simulink model "Engine_harness_model"  (R2021a)
settings: Solver=daessc  StartTime=0.0  StopTime=60*10  RelTol=1e-3  AbsTol=1e-3
PreLoadFcn:
  | Engine_harness_setup
undefined symbols (not defined in the file): engine
libraries: fl_lib x7, nesl_utility x5
settings Model: Creator=isaacito  LastModifiedBy=isaacito
settings DataIOCC: ReturnWorkspaceOutputs=off
settings DebuggingCC: UnconnectedInputMsg=none  UnconnectedOutputMsg=none  UnconnectedLineMsg=none
settings RTWCC: DLArmComputeVersion=20.02.1
settings SimscapeCC: SimscapeLogType=all  SimscapeLogSimulationStatistics=on  SimscapeLogLimitData=off

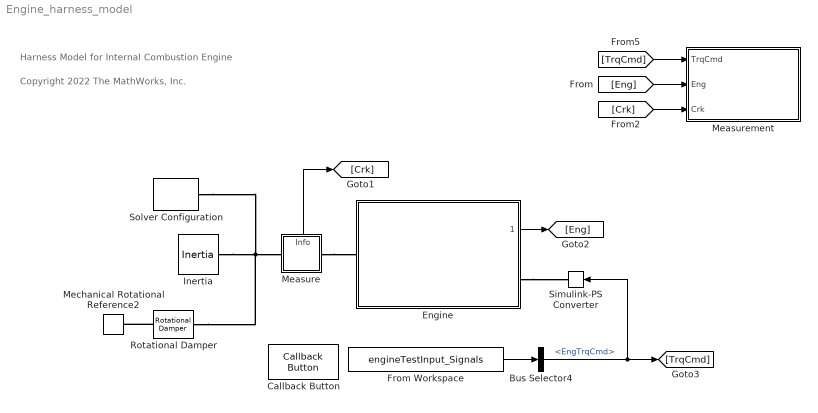
== system Engine_harness_model ==
  note: Copyright 2022 The MathWorks, Inc.
  note: Harness Model for Internal Combustion Engine
  Bus Selector4 : BusSelector  OutputSignals=EngTrqCmd
  Callback Button : CallbackButton  ButtonText=Plot input
      settings: ClickFcn="Engine_plot_inputs_simple(\"engineTestInput_Signals\")"
  Engine : Subsystem  ReferencedSubsystem=EngineCustom_refsub
  From Workspace : FromWorkspace  VariableName=engineTestInput_Signals  OutDataTypeStr=Bus: engineTestInput_Bus  OutputAfterFinalValue=Holding final value
      settings: AttributesFormatString=|
      | %<OutDataTypeStr>
      | Interpolate: %<Interpolate>
  Inertia : fl_lib/Mechanical/Rotational Elements/Inertia  inertia=engine.inertia_kg_m2 kg*m^2  num_ports=foundation.enum.numPorts2.one  w_specify=on  w_priority=High  w=initial.engine_speed_rpm rpm  w_nominal_specify=off  w_nominal_unit=rad/s  w_nominal_value=1  t_specify=off  t_priority=None  t=0 N*m  t_nominal_specify=off  t_nominal_unit=N*m  t_nominal_value=1
      settings: SourceProductBaseCode=PW,SS,VE
      settings: AttributesFormatString=|
      | Initial: %<w> [%<w_unit>]
      | Priority: %<w_priority>
  Measure : Subsystem
      settings: PortSchema="{\"entries\":[{\"content\":{\"sides\":[{\"content\":{\"connectorIds\":[\"LConn1\"]},\"type\":\"ConnectorPlacement.EquallySpacedRectSide\",\"uuid\":\"07c3a1fd-7b75-413d-9cf1-ab8270959579\"},{\"content\":{\"connectorIds\":[\"RConn1\"],\"side\":\"RIGHT\"},\"type\":\"ConnectorPlacement.EquallySpacedRectSide\",\"uuid\":\"82fb53da-addd-4028-9f33-7d5a40e2d331\"},{\"content\":{\"connectorIds\":[],\"side\":\"TOP\"},\"type\":\"ConnectorPlacement.EquallySpacedRectSide\",\"uuid\":\"88b61019-5b08-4fd4-81f8-a447296a1b8b\"},{\"content\":{\"connectorIds\":[\"Out1\"],\"side\":\"BOTTOM\"},\"type\":\"ConnectorPlacement.EquallySpacedRectSide\",\"uuid\":\"d19d7c6f-4100-43ea-b025-020464ef54d5\"}]},\"type\":\"ConnectorPlacement.EquallySpacedConnector\",\"uuid\":\"a316222e-f9ce-4776-9d48-54bd569192f1\"}],\"packageUris\":[\"http://schema.mathworks.com/mf0/Connector/R2020b\"],\"version\":\"1.0\"}"
  Measurement : Subsystem
  Mechanical Rotational Reference2 : fl_lib/Mechanical/Rotational Elements/Mechanical Rotational Reference
      settings: SourceProductBaseCode=PW,SS,VE
  Rotational Damper : fl_lib/Mechanical/Rotational Elements/Rotational Damper  D=engine.damping_Nm_per_rpm m*N/rpm  w_specify=off  w_priority=None  w=0 rad/s  w_nominal_specify=off  w_nominal_unit=rad/s  w_nominal_value=1  t_specify=off  t_priority=None  t=0 N*m  t_nominal_specify=off  t_nominal_unit=N*m  t_nominal_value=1
      settings: SourceProductBaseCode=PW,SS,VE
  Simulink-PS Converter : nesl_utility/Simulink-PS Converter  PhysicalDomain=network_engine_domain  SubClassName=ps_input  LeftPortType=input  RightPortType=output  PseudoPeriodic=off  Frequencies=[]  NoiseDistribution=none  NoiseParameters=[]  Unit=N*m  AffineConversion=off  FilteringAndDerivatives=provide  SimscapeFilterOrder=1  InputFilterTimeConstant=0.001  UdotUserProvided=0
      settings: SourceProductBaseCode=SS,PW,VE
  Solver Configuration : nesl_utility/Solver Configuration  PhysicalDomain=network_engine_domain  SubClassName=solver  LeftPortType=input  RightPortType=generic  Tones=[]  Harmonics=[]  SimulateNoise=off  Profile=off  UseLocalSampling=off  EnableSwitchedLinearOptims=on  FrequencyDomain=off  UseCCode=off  RelTol=0.001  AbsTol=0.001  MinStep=1e-09  ToWorkspace=off  RevertToSquareIcSolve=off  NumHomotopyIterations=100  PhasorMode=off  PhasorModeNumHarmonics=1  DoDC=off  ResidualTolerance=1e-09  UseLocalSolver=off  LocalSolverChoice=NE_BACKWARD_EULER_ADVANCER  LocalSolverSampleTime=0.001  DoFixedCost=off  MaxNonlinIter=3  MaxModeIter=2  ComputeImpulses=off  ImpulseIterations=2  LinearAlgebra=auto  EquationFormulation=NE_TIME_EF  DelaysMemoryBudget=1024  AutomaticFiltering=on  FilteringTimeConstant=0.001  PartitionStorageMethod=AS_NEEDED  PartitionMemoryBudget=1024  PartitionMethod=ROBUST
      settings: AttributesFormatString=Local solver: %<UseLocalSolver>  SourceProductBaseCode=SS,PW,VE
  wires:
  From Workspace/1 -> Bus Selector4/1
  Bus Selector4/1 -> [TrqCmd], Simulink-PS Converter/1  "<EngTrqCmd>"
  Engine/1 -> [Eng]
  Measure/1(Info) -> [Crk]
  [TrqCmd] -> Measurement/1(TrqCmd)
  [Eng] -> Measurement/2(Eng)
  [Crk] -> Measurement/3(Crk)
  connections:
  Rotational Damper/RConn1 -- Mechanical Rotational Reference2/LConn1
  Inertia/LConn1 -- Solver Configuration/RConn1 -- Rotational Damper/LConn1 -- Measure/RConn1
  Engine/RConn1 -- Simulink-PS Converter/RConn1
  Measure/LConn1 -- Engine/LConn1

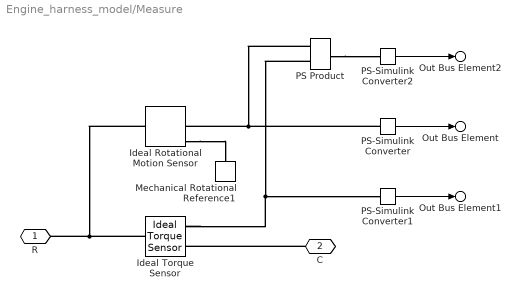
== system Engine_harness_model/Measure ==
  Ideal Rotational Motion Sensor : fl_lib/Mechanical/Mechanical Sensors/Ideal Rotational Motion Sensor  wrap_angle=simscape.enum.onoff.off  offset=0 rad
      settings: SourceProductBaseCode=PW,SS,VE
  Ideal Torque Sensor : fl_lib/Mechanical/Mechanical Sensors/Ideal Torque Sensor
      settings: SourceProductBaseCode=PW,SS,VE
  Mechanical Rotational Reference1 : fl_lib/Mechanical/Rotational Elements/Mechanical Rotational Reference
      settings: SourceProductBaseCode=PW,SS,VE
  PS Product : fl_lib/Physical Signals/Functions/PS Product
  PS-Simulink Converter : nesl_utility/PS-Simulink Converter  PhysicalDomain=network_engine_domain  SubClassName=ps_output  LeftPortType=input  RightPortType=output  PseudoPeriodic=off  Frequencies=[]  Unit=rpm  AffineConversion=off
      settings: SourceProductBaseCode=SS,PW,VE
  PS-Simulink Converter1 : nesl_utility/PS-Simulink Converter  PhysicalDomain=network_engine_domain  SubClassName=ps_output  LeftPortType=input  RightPortType=output  PseudoPeriodic=off  Frequencies=[]  Unit=N*m  AffineConversion=off
      settings: SourceProductBaseCode=SS,PW,VE
  PS-Simulink Converter2 : nesl_utility/PS-Simulink Converter  PhysicalDomain=network_engine_domain  SubClassName=ps_output  LeftPortType=input  RightPortType=output  PseudoPeriodic=off  Frequencies=[]  Unit=kW  AffineConversion=off
      settings: SourceProductBaseCode=SS,PW,VE
  R : PMIOPort  Side=Left
  C : PMIOPort  Port=2  Side=Right
  Out Bus Element : Outport  PortName=Info  Element=CrkSpd
  Out Bus Element1 : Outport  PortName=Info  Element=CrkTrq
  Out Bus Element2 : Outport  PortName=Info  Element=CrkPwr
  wires:
  PS-Simulink Converter/1 -> Out Bus Element/1
  PS-Simulink Converter1/1 -> Out Bus Element1/1
  PS-Simulink Converter2/1 -> Out Bus Element2/1
  connections:
  PS-Simulink Converter/LConn1 -- PS Product/LConn1 -- Ideal Rotational Motion Sensor/RConn2
  Ideal Rotational Motion Sensor/RConn1 -- Mechanical Rotational Reference1/LConn1
  Ideal Torque Sensor/RConn2 -- PS Product/LConn2 -- PS-Simulink Converter1/LConn1
  Ideal Torque Sensor/LConn1 -- R/RConn1 -- Ideal Rotational Motion Sensor/LConn1
  C/RConn1 -- Ideal Torque Sensor/RConn1
  PS Product/RConn1 -- PS-Simulink Converter2/LConn1

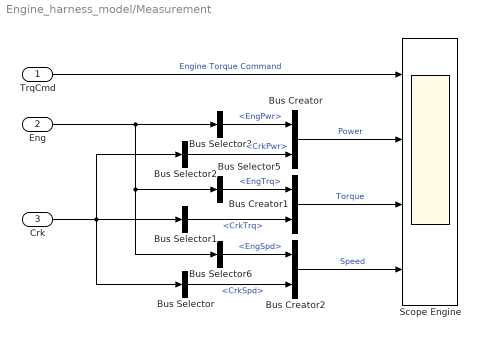
== system Engine_harness_model/Measurement ==
  TrqCmd : Inport
  Eng : Inport  Port=2
  Crk : Inport  Port=3
  Bus Creator : BusCreator  Inputs=2
  Bus Creator1 : BusCreator  Inputs=2
  Bus Creator2 : BusCreator  Inputs=2
  Bus Selector : BusSelector  OutputSignals=CrkSpd
  Bus Selector1 : BusSelector  OutputSignals=CrkTrq
  Bus Selector2 : BusSelector  OutputSignals=CrkPwr
  Bus Selector3 : BusSelector  OutputSignals=EngPwr
  Bus Selector5 : BusSelector  OutputSignals=EngTrq
  Bus Selector6 : BusSelector  OutputSignals=EngSpd
  Scope Engine : Scope  NumInputPorts=4
  wires:
  Crk/1 -> Bus Selector/1, Bus Selector2/1, Bus Selector1/1
  Bus Selector6/1 -> Bus Creator2/1  "<EngSpd>"
  Bus Selector5/1 -> Bus Creator1/1  "<EngTrq>"
  Bus Selector1/1 -> Bus Creator1/2  "<CrkTrq>"
  Eng/1 -> Bus Selector5/1, Bus Selector6/1, Bus Selector3/1
  Bus Creator1/1 -> Scope Engine/3  "Torque"
  Bus Selector2/1 -> Bus Creator/2  "<CrkPwr>"
  Bus Selector3/1 -> Bus Creator/1  "<EngPwr>"
  Bus Creator/1 -> Scope Engine/2  "Power"
  TrqCmd/1 -> Scope Engine/1  "Engine Torque Command"
  Bus Creator2/1 -> Scope Engine/4  "Speed"
  Bus Selector/1 -> Bus Creator2/2  "<CrkSpd>"
